simulink model "Plant"  (R2021a)
settings: Solver=VariableStepAuto  StartTime=0.0  StopTime=10.0  RelTol=1e-3
undefined symbols (not defined in the file): g_n, Jm, Jp, KcRa, Km, L_n, M_n, N_n, T_ba_n, x0
libraries: simulink x1, simulink_extras x1
settings Model: Creator=domin  LastModifiedBy=domin
settings ModelReferenceCC: ModelReferenceNumInstancesAllowed=Single

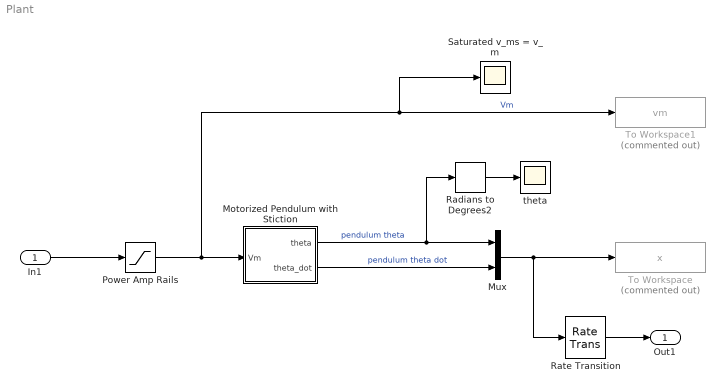
== system Plant ==
  In1 : Inport
  Motorized Pendulum with Stiction : Subsystem
  Mux : Mux  Inputs=2
  Power Amp Rails : Saturate  UpperLimit=15  LowerLimit=-15
  Radians to Degrees2 : simulink_extras/Transformations/Radians to Degrees
  Rate Transition : RateTransition  OutPortSampleTime=0.01
  Saturated v_ms = v_m : Scope
  To Workspace : ToWorkspace  Commented=on  VariableName=x  SampleTime=-1
  To Workspace1 : ToWorkspace  Commented=on  VariableName=vm
  theta : Scope
  Out1 : Outport
  wires:
  Radians to Degrees2/1 -> theta/1
  Motorized Pendulum with Stiction/2(theta_dot) -> Mux/2  "pendulum theta dot"
  Motorized Pendulum with Stiction/1(theta) -> Radians to Degrees2/1, Mux/1  "pendulum theta"
  Mux/1 -> Rate Transition/1, To Workspace/1
  Power Amp Rails/1 -> Saturated v_ms = v_m/1, To Workspace1/1, Motorized Pendulum with Stiction/1(Vm)  "Vm"
  In1/1 -> Power Amp Rails/1
  Rate Transition/1 -> Out1/1

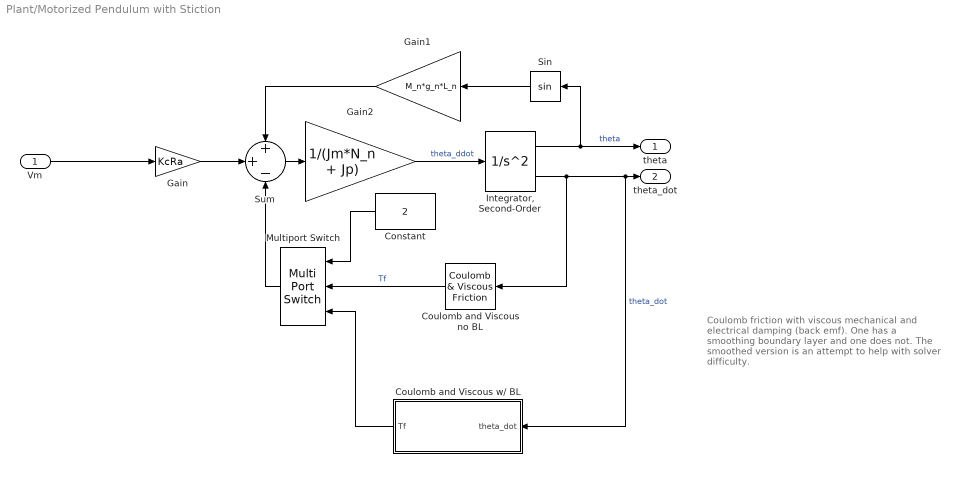
== system Plant/Motorized Pendulum with Stiction ==
  note: Coulomb friction with viscous mechanical
      | and electrical damping (back emf). One has a
      | smoothing boundary layer and one does not.
      | The smoothed version is an attempt to help with
      | solver difficulty.
  Vm : Inport
  Constant : Constant  Value=2
  Coulomb and Viscous no BL : simulink/Discontinuities/Coulomb & Viscous Friction  offset=T_ba_n  gain=N_n*KcRa/Km
  Coulomb and Viscous w/ BL : MATLAB Function  TreatAsAtomicUnit=on
  Gain : Gain  Gain=KcRa
  Gain1 : Gain  Gain=M_n*g_n*L_n
  Gain2 : Gain  Gain=1/(Jm*N_n + Jp)
  "Integrator, Second-Order" : SecondOrderIntegrator  ICX=x0(1)  ICDXDT=x0(2)  ZeroCross=off
  Multiport Switch : MultiPortSwitch  Inputs=2
  Sin : Trigonometry
  Sum : Sum  Inputs=++-
  theta : Outport
  theta_dot : Outport  Port=2
  wires:
  Gain2/1 -> "Integrator, Second-Order"/1  "theta_ddot"
  Sin/1 -> Gain1/1
  "Integrator, Second-Order"/2 -> Coulomb and Viscous w/ BL/1(theta_dot), theta_dot/1, Coulomb and Viscous no BL/1  "theta_dot"
  "Integrator, Second-Order"/1 -> Sin/1, theta/1  "theta"
  Gain1/1 -> Sum/1
  Sum/1 -> Gain2/1
  Vm/1 -> Gain/1
  Gain/1 -> Sum/2
  Constant/1 -> Multiport Switch/1
  Multiport Switch/1 -> Sum/3
  Coulomb and Viscous w/ BL/1(Tf) -> Multiport Switch/3
  Coulomb and Viscous no BL/1 -> Multiport Switch/2  "Tf"

== matlab function Plant/Motorized Pendulum with Stiction/Coulomb and Viscous w// BL ==
  data: theta_dot input; Tf output; Km parameter; KcRa parameter; N_n parameter; T_ba_n parameter
function Tf = fcn(theta_dot, Km,  KcRa, N_n, T_ba_n)

Tf = N_n*KcRa/Km*theta_dot + T_ba_n*erf(1e6*theta_dot);
